simulink model "Stateflow_Traffic"  (R2016a)
settings: Solver=FixedStepDiscrete  StartTime=0.0  StopTime=15  RelTol=1e-3
libraries: simulink x1
settings Model: Creator=Mohamed Fawzy  LastModifiedBy=Mohamed Fawzy
settings OptimizationCC: DefaultParameterBehavior=Inlined  OptimizeModelRefInitCode=on  LifeSpan=1
settings RTWCC: SystemTargetFile=ert.tlc  GenCodeOnly=on  GenerateMakefile=off  TemplateMakefile=ert_default_tmf  GenerateReport=on  IncludeHyperlinkInReport=on  LaunchReport=on  GenerateTraceInfo=on  GenerateTraceReport=on  GenerateTraceReportSl=on  GenerateTraceReportSf=on  GenerateTraceReportEml=on
settings CodeAppCC: ForceParamTrailComments=on  IgnoreCustomStorageClasses=off  OperatorAnnotations=on  SimulinkDataObjDesc=on  SFDataObjDesc=on  MATLABFcnDesc=on  InsertBlockDesc=on  MATLABSourceComments=on
settings ERTTargetCC: GenerateSampleERTMain=on  SuppressErrorStatus=on  InlinedParameterPlacement=NonHierarchical  ERTCustomFileTemplate=example_file_process.tlc

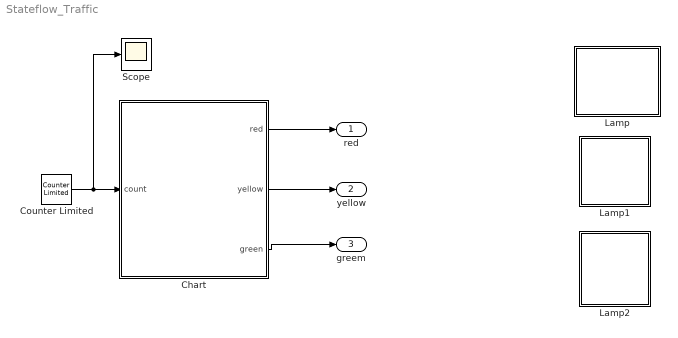
== system Stateflow_Traffic ==
  Chart : Stateflow chart  TreatAsAtomicUnit=on
  Counter Limited : simulink/Sources/Counter Limited  uplimit=15  tsamp=1
  Lamp : Subsystem  DialogController=hmiCreateDDGDialog  IsWebBlock=on  mask(MWDashboardBlock){webBlockId=73115a94-b972-4f88-bb2c-e64ed945614e, webBlockType=lamp, ShowInLibBrowser=on, ShowInitialText=on, HMISrcModelName=Stateflow_Traffic}
      mask prompts: webBlockType "WebBlock Type"; HMISrcModelName "Source Model"
      mask Help: helpview([docroot '/mapfiles/simulink.map'], 'hmi_lamp')
      mask Display:
      | if strcmp(get_param(bdroot(gcb),'BlockDiagramType'), 'library')
      |     image([(matlabroot) '/toolbox/simulink/hmi/icons/Lamp.png']);
      | end
  Lamp1 : Subsystem  DialogController=hmiCreateDDGDialog  IsWebBlock=on  mask(MWDashboardBlock){webBlockId=9d45d177-c927-4783-9c35-82a52a8fd86d, webBlockType=lamp, ShowInLibBrowser=on, ShowInitialText=on, HMISrcModelName=Stateflow_Traffic}
      mask prompts: webBlockType "WebBlock Type"; HMISrcModelName "Source Model"
      mask Help: helpview([docroot '/mapfiles/simulink.map'], 'hmi_lamp')
      mask Display:
      | if strcmp(get_param(bdroot(gcb),'BlockDiagramType'), 'library')
      |     image([(matlabroot) '/toolbox/simulink/hmi/icons/Lamp.png']);
      | end
  Lamp2 : Subsystem  DialogController=hmiCreateDDGDialog  IsWebBlock=on  mask(MWDashboardBlock){webBlockId=f7dd5391-e987-4971-8a8c-d5fb5b6815e6, webBlockType=lamp, ShowInLibBrowser=on, ShowInitialText=on, HMISrcModelName=Stateflow_Traffic}
      mask prompts: webBlockType "WebBlock Type"; HMISrcModelName "Source Model"
      mask Help: helpview([docroot '/mapfiles/simulink.map'], 'hmi_lamp')
      mask Display:
      | if strcmp(get_param(bdroot(gcb),'BlockDiagramType'), 'library')
      |     image([(matlabroot) '/toolbox/simulink/hmi/icons/Lamp.png']);
      | end
  Scope : Scope
  red : Outport
  "yellow " : Outport  Port=2
  "greem " : Outport  Port=3
  wires:
  Chart/1(red) -> red/1
  Chart/2(yellow) -> "yellow "/1
  Chart/3(green) -> "greem "/1
  Counter Limited/1 -> Scope/1, Chart/1(count)

== system Stateflow_Traffic/Lamp ==

== system Stateflow_Traffic/Lamp1 ==

== system Stateflow_Traffic/Lamp2 ==

== stateflow chart Stateflow_Traffic/Chart ==
  state counter
    en:
    du:
    ex:
    state Stop
      en:
      red=1;
      du:
      red=1;
      ex:
      red=0;
    state Hold
      en:
      yellow=1;
      du:
      yellow=1;
      ex:
      yellow=0;
    state GO
      en:
      green=1;
      du:
      green=1;
      ex:
      green=0;
    (default) -> Stop
    Stop -> Hold : [count==3]
    Hold -> GO [order 1] : [count==6]
    GO -> Hold : [count ==9]
    Hold -> Stop [order 2] : [count==12]
  (default) -> counter
  data: red output boolean; yellow output boolean; green output boolean; count input uint8
